simulink model "Single Phase Induction Motor with all methods (final)"  (R2023b)
settings: Solver=ode23s  StartTime=0.0  StopTime=10.0  MaxStep=1e-4  RelTol=1e-3
undefined symbols (not defined in the file): Capacitor, Run, Start
libraries: spsIGBTDiodeLib x12, simulink x9, spsDCVoltageSourceLib x3, spsRMSLib x3, spsSinglePhaseAsynchronousMachineLib x3, spsVoltageMeasurementLib x3, slpidlib x2, spspowerguiLib x2, spsControlledVoltageSourceLib x1, sps_lib x1
settings Model: Creator=Haier  LastModifiedBy=Haier

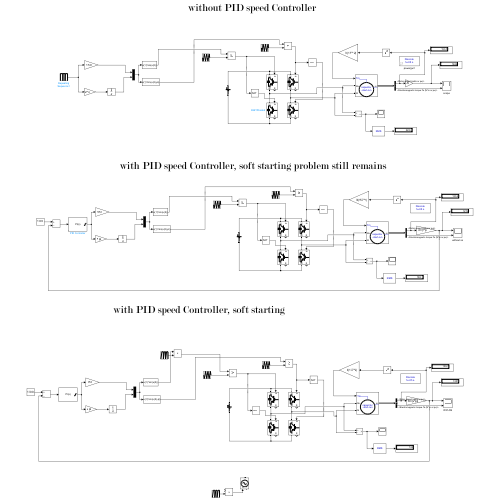
[thumbnail: Simulink's stored preview of the top-level diagram]
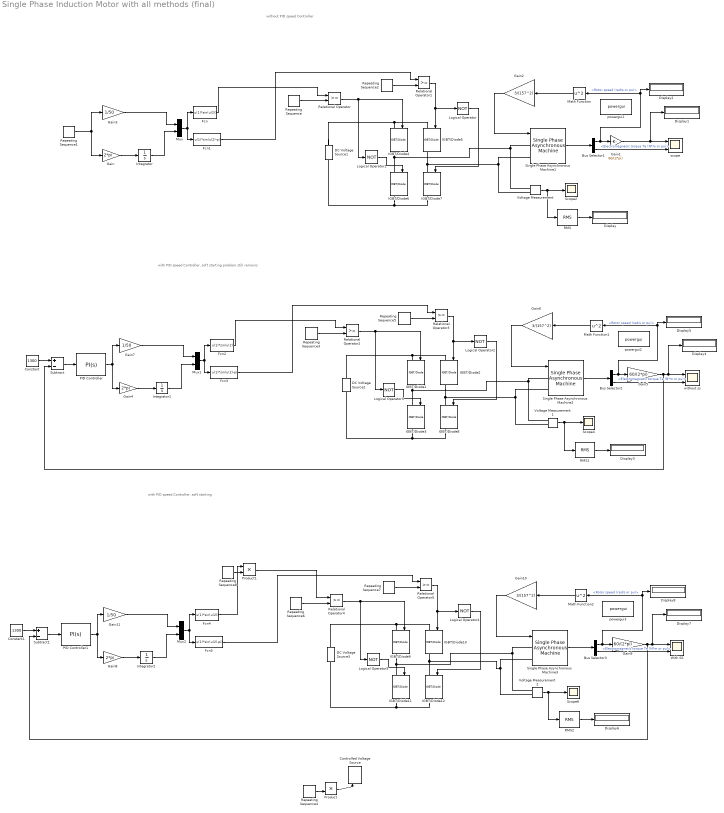
== system Single Phase Induction Motor with all methods (final) ==
  note: without PID speed Controller
  note: with PID speed Controller, soft starting problem still remains
  note: with PID speed Controller, soft starting
  Bus Selector1 : BusSelector  OutputSignals=Mechanical.Rotor speed (rad/s or pu),Mechanical.Electromagnetic torque Te (N*m or pu)
  Bus Selector2 : BusSelector  OutputSignals=Mechanical.Rotor speed (rad/s or pu),Mechanical.Electromagnetic torque Te (N*m or pu)
  Bus Selector3 : BusSelector  OutputSignals=Mechanical.Rotor speed (rad/s or pu),Mechanical.Electromagnetic torque Te (N*m or pu)
  Constant : Constant  Value=1300
  Constant1 : Constant  Value=1300
  Controlled Voltage Source : spsControlledVoltageSourceLib/Controlled Voltage Source  Initialize=on  Source_Type=AC  Amplitude=0  Phase=0  Frequency=0  Measurements=None
  DC Voltage Source1 : spsDCVoltageSourceLib/DC Voltage Source  Amplitude=325  Measurements=None
  DC Voltage Source2 : spsDCVoltageSourceLib/DC Voltage Source  Amplitude=325  Measurements=None
  DC Voltage Source3 : spsDCVoltageSourceLib/DC Voltage Source  Amplitude=325  Measurements=None
  Display{,1..8} (9 alike) : Display
  Fcn : Fcn  Expr=u(1)*sin(u(2))
  Fcn1 : Fcn  Expr=u(1)*sin(u(2)-pi)
  Fcn2 : Fcn  Expr=u(1)*sin(u(2))
  Fcn3 : Fcn  Expr=u(1)*sin(u(2)-pi)
  Fcn4 : Fcn  Expr=u(1)*sin(u(2))
  Fcn5 : Fcn  Expr=u(1)*sin(u(2)-pi)
  Gain : Gain  Gain=2*pi
  Gain1 : Gain  Gain=60/(2*pi)
  Gain10 : Gain  Gain=3/(157^2)
  Gain11 : Gain  Gain=1/50
  Gain2 : Gain  Gain=3/(157^2)
  Gain3 : Gain  Gain=1/50
  Gain4 : Gain  Gain=2*pi
  Gain5 : Gain  Gain=60/(2*pi)
  Gain6 : Gain  Gain=3/(157^2)
  Gain7 : Gain  Gain=1/50
  Gain8 : Gain  Gain=2*pi
  Gain9 : Gain  Gain=60/(2*pi)
  IGBT/Diode{1..12} (12 alike) : spsIGBTDiodeLib/IGBT//Diode  Ron=1e-3  Rs=1e5  Cs=inf  Measurements=on
  Integrator : Integrator
  Integrator1 : Integrator
  Integrator2 : Integrator
  Logical Operator{,1..5} (6 alike) : Logic  Operator=NOT  AllPortsSameDT=off  OutDataTypeStr=boolean
  Math Function : Math  Operator=square
  Math Function1 : Math  Operator=square
  Math Function2 : Math  Operator=square
  Mux : Mux  Inputs=2
  Mux1 : Mux  Inputs=2
  Mux2 : Mux  Inputs=2
  PID Controller : slpidlib/PID Controller  Controller=PI  Form=Parallel  TimeDomain=Continuous-time  UseExternalTs=off  SampleTime=-1  IntegratorMethod=Forward Euler  FilterMethod=Forward Euler  ControllerParametersSource=internal  P=0.00001  I=0.09  UseKiTs=off  D=0  N=100  UseFilter=on  TunerSelectOption=Transfer Function Based (PID Tuner App)  InitialConditionSource=internal  InitialConditionForIntegrator=0  InitialConditionForFilter=0  DifferentiatorICPrevScaledInput=0  ExternalReset=none  TrackingMode=off  Kt=1  LimitOutput=on  SatLimitsSource=internal  UpperSaturationLimit=50  LowerSaturationLimit=-50  LinearizeAsGain=on  AntiWindupMode=clamping  Kb=1  LimitIntegrator=off  UpperIntegratorSaturationLimit=inf  LowerIntegratorSaturationLimit=-inf  POutMin=[]  POutMax=[]  IOutMin=[]  IOutMax=[]  DOutMin=[]  DOutMax=[]  NOutMin=[]  NOutMax=[]  SumOutMin=[]  SumOutMax=[]  SaturationOutMin=[]  SaturationOutMax=[]  PParamMin=[]  PParamMax=[]  IParamMin=[]  IParamMax=[]  DParamMin=[]  DParamMax=[]  NParamMin=[]  NParamMax=[]  KbParamMin=[]  KbParamMax=[]  KtParamMin=[]  KtParamMax=[]  KbOutMin=[]  KbOutMax=[]  KtOutMin=[]  KtOutMax=[]  IntegratorOutMin=[]  IntegratorOutMax=[]  FilterOutMin=[]  FilterOutMax=[]  SumI1OutMin=[]  SumI1OutMax=[]  SumI2OutMin=[]  SumI2OutMax=[]  SumI3OutMin=[]  SumI3OutMax=[]  SumI4OutMin=[]  SumI4OutMax=[]  SumDOutMin=[]  SumDOutMax=[]  DifferentiatorOutMin=[]  DifferentiatorOutMax=[]  FilterDiffOutCoefMin=[]  FilterDiffOutCoefMax=[]  ReciprocalOutMin=[]  ReciprocalOutMax=[]  SumDenOutMin=[]  SumDenOutMax=[]  SumNumOutMin=[]  SumNumOutMax=[]  DivideOutMin=[]  DivideOutMax=[]  UdiffTsProdOutMin=[]  UdiffTsProdOutMax=[]  NTsProdOutMin=[]  NTsProdOutMax=[]  UintegralTsProdOutMin=[]  UintegralTsProdOutMax=[]  UngainTsProdOutMin=[]  UngainTsProdOutMax=[]  ClampingZeroOutDataTypeStr=Inherit: Inherit via back propagation  ClampingZeroOutMin=[]  ClampingZeroOutMax=[]  FilterDenConstantOutDataTypeStr=Inherit: Inherit via back propagation  FilterDenConstantOutMin=[]  FilterDenConstantOutMax=[]  PCopyOutDataTypeStr=Inherit: Inherit via back propagation  PCopyOutMin=[]  PCopyOutMax=[]  NCopyOutDataTypeStr=Inherit: Inherit via back propagation  NCopyOutMin=[]  NCopyOutMax=[]  IntegratorContinuousStateAttributes=''  IntegratorStateMustResolveToSignalObject=off  IntegratorRTWStateStorageClass=Auto  FilterContinuousStateAttributes=''  FilterStateMustResolveToSignalObject=off  FilterRTWStateStorageClass=Auto  ParallelPVariant=InternalParameters  IdealPVariant=Disabled  IVariant=InternalParameters  DVariant=Disabled  IntegratorVariant=Continuous  SatVariant=Enabled  AWVariant=ContClampingParallel  PCopyVariant=Disabled  TRVariant=Disabled  FdbkBlocksVariant=Forward  IdealPFdbkVariant=Disabled  SatFdbkVariant=Disabled  DerivativeFilterVariant=Disabled  NVariant=Disabled  NCopyVariant=Disabled_SignalSpec  FilterICVariant=Disabled  IntegratorICVariant=InternalICs  ExternalResetVariant=Disabled  TRSumVariant=Passthrough  SumFdbkVariant=Disabled  SumVariant=Sum_PI  TsampFilterVariant=InternalTs  TsampNgainVariant=Passthrough  TsampIntegralVariant=Disabled_SignalSpec  ExternalSaturationOutDataTypeStr=Inherit: Same as second input
  PID Controller1 : slpidlib/PID Controller  Controller=PI  Form=Parallel  TimeDomain=Continuous-time  UseExternalTs=off  SampleTime=-1  IntegratorMethod=Forward Euler  FilterMethod=Forward Euler  ControllerParametersSource=internal  P=0.00001  I=0.09  UseKiTs=off  D=0  N=100  UseFilter=on  TunerSelectOption=Transfer Function Based (PID Tuner App)  InitialConditionSource=internal  InitialConditionForIntegrator=0  InitialConditionForFilter=0  DifferentiatorICPrevScaledInput=0  ExternalReset=none  TrackingMode=off  Kt=1  LimitOutput=on  SatLimitsSource=internal  UpperSaturationLimit=50  LowerSaturationLimit=-50  LinearizeAsGain=on  AntiWindupMode=clamping  Kb=1  LimitIntegrator=off  UpperIntegratorSaturationLimit=inf  LowerIntegratorSaturationLimit=-inf  POutMin=[]  POutMax=[]  IOutMin=[]  IOutMax=[]  DOutMin=[]  DOutMax=[]  NOutMin=[]  NOutMax=[]  SumOutMin=[]  SumOutMax=[]  SaturationOutMin=[]  SaturationOutMax=[]  PParamMin=[]  PParamMax=[]  IParamMin=[]  IParamMax=[]  DParamMin=[]  DParamMax=[]  NParamMin=[]  NParamMax=[]  KbParamMin=[]  KbParamMax=[]  KtParamMin=[]  KtParamMax=[]  KbOutMin=[]  KbOutMax=[]  KtOutMin=[]  KtOutMax=[]  IntegratorOutMin=[]  IntegratorOutMax=[]  FilterOutMin=[]  FilterOutMax=[]  SumI1OutMin=[]  SumI1OutMax=[]  SumI2OutMin=[]  SumI2OutMax=[]  SumI3OutMin=[]  SumI3OutMax=[]  SumI4OutMin=[]  SumI4OutMax=[]  SumDOutMin=[]  SumDOutMax=[]  DifferentiatorOutMin=[]  DifferentiatorOutMax=[]  FilterDiffOutCoefMin=[]  FilterDiffOutCoefMax=[]  ReciprocalOutMin=[]  ReciprocalOutMax=[]  SumDenOutMin=[]  SumDenOutMax=[]  SumNumOutMin=[]  SumNumOutMax=[]  DivideOutMin=[]  DivideOutMax=[]  UdiffTsProdOutMin=[]  UdiffTsProdOutMax=[]  NTsProdOutMin=[]  NTsProdOutMax=[]  UintegralTsProdOutMin=[]  UintegralTsProdOutMax=[]  UngainTsProdOutMin=[]  UngainTsProdOutMax=[]  ClampingZeroOutDataTypeStr=Inherit: Inherit via back propagation  ClampingZeroOutMin=[]  ClampingZeroOutMax=[]  FilterDenConstantOutDataTypeStr=Inherit: Inherit via back propagation  FilterDenConstantOutMin=[]  FilterDenConstantOutMax=[]  PCopyOutDataTypeStr=Inherit: Inherit via back propagation  PCopyOutMin=[]  PCopyOutMax=[]  NCopyOutDataTypeStr=Inherit: Inherit via back propagation  NCopyOutMin=[]  NCopyOutMax=[]  IntegratorContinuousStateAttributes=''  IntegratorStateMustResolveToSignalObject=off  IntegratorRTWStateStorageClass=Auto  FilterContinuousStateAttributes=''  FilterStateMustResolveToSignalObject=off  FilterRTWStateStorageClass=Auto  ParallelPVariant=InternalParameters  IdealPVariant=Disabled  IVariant=InternalParameters  DVariant=Disabled  IntegratorVariant=Continuous  SatVariant=Enabled  AWVariant=ContClampingParallel  PCopyVariant=Disabled  TRVariant=Disabled  FdbkBlocksVariant=Forward  IdealPFdbkVariant=Disabled  SatFdbkVariant=Disabled  DerivativeFilterVariant=Disabled  NVariant=Disabled  NCopyVariant=Disabled_SignalSpec  FilterICVariant=Disabled  IntegratorICVariant=InternalICs  ExternalResetVariant=Disabled  TRSumVariant=Passthrough  SumFdbkVariant=Disabled  SumVariant=Sum_PI  TsampFilterVariant=InternalTs  TsampNgainVariant=Passthrough  TsampIntegralVariant=Disabled_SignalSpec  ExternalSaturationOutDataTypeStr=Inherit: Same as second input
  Product : Product
  Product1 : Product
  RMS : spsRMSLib/RMS  TrueRMS=off  Freq=50  RMSInit=0  Ts=0
  RMS1 : spsRMSLib/RMS  TrueRMS=off  Freq=50  RMSInit=0  Ts=0
  RMS2 : spsRMSLib/RMS  TrueRMS=off  Freq=50  RMSInit=0  Ts=0
  Relational Operator{,1..5} (6 alike) : RelationalOperator  OutDataTypeStr=boolean  RndMeth=Simplest  InputSameDT=off
  Repeating Sequence{,2..3,5..7} (6 alike) : simulink/Sources/Repeating Sequence  rep_seq_t=[0 0.25/5000 0.5/5000 0.75/5000 1/5000]  rep_seq_y=[0 -1 0 1 0]
  Repeating Sequence1 : simulink/Sources/Repeating Sequence  rep_seq_t=[0 0.2 10]  rep_seq_y=[0 50 50]
  Repeating Sequence4 : simulink/Sources/Repeating Sequence  rep_seq_t=[0 4 10]  rep_seq_y=[0 1 1]
  Repeating Sequence8 : simulink/Sources/Repeating Sequence  rep_seq_t=[0 4 10]  rep_seq_y=[0 1 1]
  Scope2 : Scope
  Scope4 : Scope
  Scope6 : Scope
  Single Phase Asynchronous Machine1 : spsSinglePhaseAsynchronousMachineLib/Single Phase Asynchronous Machine  MechanicalLoad=Torque Tm  UNITS=SI  MachineType=Capacitor-Start-Run  MeasurementBus=off  NominalParameters="[ .25*746  220  50]"  MainWindingStator="[2.02  7.4e-3]"  MainWindingRotor="[4.12  5.6e-3]"  MutualInductance=0.1772  AuxiliaryWinding="[7.14  8.5e-3]"  Mechanical="[0.0146  0  2 1.18]"  CapacitorStart="[2  254.7e-6]"  CapacitorRun="[18  21.1e-6]"  DisconnectionSpeed=75  InitialSpeed=0  DataType=SI  TsPowergui=0  TsBlock=-1
      settings: LibrarySourceBlock=|
      | sps_lib/Electrical Machines/Single Phase
      | Asynchronous Machine
  Single Phase Asynchronous Machine2 : spsSinglePhaseAsynchronousMachineLib/Single Phase Asynchronous Machine  MechanicalLoad=Torque Tm  UNITS=SI  MachineType=Capacitor-Start-Run  MeasurementBus=off  NominalParameters="[ .25*746  220  50]"  MainWindingStator="[2.02  7.4e-3]"  MainWindingRotor="[4.12  5.6e-3]"  MutualInductance=0.1772  AuxiliaryWinding="[7.14  8.5e-3]"  Mechanical="[0.0146  0  2 1.18]"  CapacitorStart="[2  254.7e-6]"  CapacitorRun="[18  21.1e-6]"  DisconnectionSpeed=75  InitialSpeed=0  DataType=SI  TsPowergui=0  TsBlock=-1
      settings: LibrarySourceBlock=|
      | sps_lib/Electrical Machines/Single Phase
      | Asynchronous Machine
  Single Phase Asynchronous Machine3 : spsSinglePhaseAsynchronousMachineLib/Single Phase Asynchronous Machine  MechanicalLoad=Torque Tm  UNITS=SI  MachineType=Capacitor-Start-Run  MeasurementBus=off  NominalParameters="[ .25*746  220  50]"  MainWindingStator="[2.02  7.4e-3]"  MainWindingRotor="[4.12  5.6e-3]"  MutualInductance=0.1772  AuxiliaryWinding="[7.14  8.5e-3]"  Mechanical="[0.0146  0  2 1.18]"  CapacitorStart="[2  254.7e-6]"  CapacitorRun="[18  21.1e-6]"  DisconnectionSpeed=75  InitialSpeed=0  DataType=SI  TsPowergui=0  TsBlock=-1
      settings: LibrarySourceBlock=|
      | sps_lib/Electrical Machines/Single Phase
      | Asynchronous Machine
  Subtract : Sum  Inputs=+-
  Subtract1 : Sum  Inputs=+-
  Voltage Measurement : spsVoltageMeasurementLib/Voltage Measurement  PhasorSimulation=off  OutputType=Complex  PSBequivalent=0
  Voltage Measurement1 : spsVoltageMeasurementLib/Voltage Measurement  PhasorSimulation=off  OutputType=Complex  PSBequivalent=0
  Voltage Measurement2 : spsVoltageMeasurementLib/Voltage Measurement  PhasorSimulation=off  OutputType=Complex  PSBequivalent=0
  With SS : Scope  NumInputPorts=2
  powergui1 : sps_lib/powergui  Priority=1  SimulationMode=Discrete  SampleTime=1e-5  frequency=60  Iterations=50  frequencyindice=0  Pbase=100e6  ErrMax=1e-4  UnitsV=kV  UnitsW=MW  buscounter=0  FunctionMessages=off  echomessages=off  EnableUseOfTLC=off  CurrentSourceSwitches=off  DisableSnubberDevices=off  DisableRonSwitches=off  DisableVfSwitches=off  DisplayEquations=off  AutomaticDiscreteSolvers=off  SolverType=Tustin/Backward Euler (TBE)  Interpol=off  ExternalGateDelay=off  methode=off  Ts=100  x0status=blocks  SPID=on  SwTol=0  HookPort=off  NonlinearTolerance=1e-4  nMaxIteration=100  ContinueOnMaxIteration=off  RestoreLinks=warning  ResistiveCurrentMeasurement=off  Frange=[0:2:500]  Ylog=off  Xlog=on  ShowGrid=off  save=off  variable=ZData  structure=0  ZoomFFT=off  StartTime=0.0  cycles=1  DisplayStyle=1  fundamental=60  FreqAxis=off  MaxFrequency=1000  frequencyindicesteady=1  RmsSteady=1  display=off
  powergui2 : spspowerguiLib/powergui  Priority=1  SimulationMode=Discrete  SampleTime=1e-5  frequency=60  Iterations=50  frequencyindice=0  Pbase=100e6  ErrMax=1e-4  UnitsV=kV  UnitsW=MW  buscounter=0  FunctionMessages=off  echomessages=off  EnableUseOfTLC=off  CurrentSourceSwitches=off  DisableSnubberDevices=off  DisableRonSwitches=off  DisableVfSwitches=off  DisplayEquations=off  AutomaticDiscreteSolvers=off  SolverType=Tustin/Backward Euler (TBE)  Interpol=off  ExternalGateDelay=off  methode=off  Ts=100  x0status=blocks  SPID=on  SwTol=0  HookPort=off  NonlinearTolerance=1e-4  nMaxIteration=100  ContinueOnMaxIteration=off  RestoreLinks=warning  ResistiveCurrentMeasurement=off  Frange=[0:2:500]  Ylog=off  Xlog=on  ShowGrid=off  save=off  variable=ZData  structure=0  ZoomFFT=off  StartTime=0.0  cycles=1  DisplayStyle=1  fundamental=60  FreqAxis=off  MaxFrequency=1000  frequencyindicesteady=1  RmsSteady=1  display=off
  powergui3 : spspowerguiLib/powergui  Priority=1  SimulationMode=Discrete  SampleTime=1e-5  frequency=60  Iterations=50  frequencyindice=0  Pbase=100e6  ErrMax=1e-4  UnitsV=kV  UnitsW=MW  buscounter=0  FunctionMessages=off  echomessages=off  EnableUseOfTLC=off  CurrentSourceSwitches=off  DisableSnubberDevices=off  DisableRonSwitches=off  DisableVfSwitches=off  DisplayEquations=off  AutomaticDiscreteSolvers=off  SolverType=Tustin/Backward Euler (TBE)  Interpol=off  ExternalGateDelay=off  methode=off  Ts=100  x0status=blocks  SPID=on  SwTol=0  HookPort=off  NonlinearTolerance=1e-4  nMaxIteration=100  ContinueOnMaxIteration=off  RestoreLinks=warning  ResistiveCurrentMeasurement=off  Frange=[0:2:500]  Ylog=off  Xlog=on  ShowGrid=off  save=off  variable=ZData  structure=0  ZoomFFT=off  StartTime=0.0  cycles=1  DisplayStyle=1  fundamental=60  FreqAxis=off  MaxFrequency=1000  frequencyindicesteady=1  RmsSteady=1  display=off
  scope : Scope  NumInputPorts=2
  without ss : Scope  NumInputPorts=2
  wires:
  Bus Selector1/1 -> Math Function/1, Display2/1, Gain1/1  "<Rotor speed (rad/s or pu)>"
  Voltage Measurement/1 -> RMS/1, Scope2/1
  Gain1/1 -> Display1/1, scope/1
  Math Function/1 -> Gain2/1
  Gain2/1 -> Single Phase Asynchronous Machine1/1
  Single Phase Asynchronous Machine1/1 -> Bus Selector1/1
  Bus Selector1/2 -> scope/2  "<Electromagnetic torque Te (N*m or pu)>"
  Integrator/1 -> Mux/2
  Gain3/1 -> Mux/1
  Mux/1 -> Fcn1/1, Fcn/1
  Gain/1 -> Integrator/1
  Repeating Sequence1/1 -> Gain/1, Gain3/1
  RMS/1 -> Display/1
  Relational Operator1/1 -> IGBT/Diode5/1, Logical Operator/1
  Relational Operator/1 -> Logical Operator1/1, IGBT/Diode4/1
  Logical Operator1/1 -> IGBT/Diode6/1
  Logical Operator/1 -> IGBT/Diode7/1
  Repeating Sequence/1 -> Relational Operator/2
  Repeating Sequence2/1 -> Relational Operator1/2
  Fcn/1 -> Relational Operator/1
  Fcn1/1 -> Relational Operator1/1
  Gain4/1 -> Integrator1/1
  Integrator1/1 -> Mux1/2
  Repeating Sequence5/1 -> Relational Operator3/2
  Relational Operator3/1 -> IGBT/Diode2/1, Logical Operator2/1
  Fcn2/1 -> Relational Operator2/1
  Fcn3/1 -> Relational Operator3/1
  Logical Operator3/1 -> IGBT/Diode3/1
  Gain7/1 -> Mux1/1
  Relational Operator2/1 -> Logical Operator3/1, IGBT/Diode1/1
  Repeating Sequence3/1 -> Relational Operator2/2
  Mux1/1 -> Fcn3/1, Fcn2/1
  Gain6/1 -> Single Phase Asynchronous Machine2/1
  Single Phase Asynchronous Machine2/1 -> Bus Selector2/1
  Math Function1/1 -> Gain6/1
  Voltage Measurement1/1 -> RMS1/1, Scope4/1
  Bus Selector2/1 -> Math Function1/1, Display5/1, Gain5/1  "<Rotor speed (rad/s or pu)>"
  Bus Selector2/2 -> without ss/2  "<Electromagnetic torque Te (N*m or pu)>"
  RMS1/1 -> Display3/1
  Logical Operator2/1 -> IGBT/Diode8/1
  Constant/1 -> Subtract/1
  Gain5/1 -> Subtract/2, Display4/1, without ss/1
  PID Controller/1 -> Gain4/1, Gain7/1
  Subtract/1 -> PID Controller/1
  Subtract1/1 -> PID Controller1/1
  Bus Selector3/1 -> Math Function2/1, Display8/1, Gain9/1  "<Rotor speed (rad/s or pu)>"
  Math Function2/1 -> Gain10/1
  Single Phase Asynchronous Machine3/1 -> Bus Selector3/1
  Bus Selector3/2 -> With SS/2  "<Electromagnetic torque Te (N*m or pu)>"
  Mux2/1 -> Fcn5/1, Fcn4/1
  Relational Operator4/1 -> Logical Operator5/1, IGBT/Diode9/1
  Logical Operator5/1 -> IGBT/Diode11/1
  Fcn5/1 -> Relational Operator5/1
  Gain11/1 -> Mux2/1
  Relational Operator5/1 -> IGBT/Diode10/1, Logical Operator4/1
  Repeating Sequence6/1 -> Relational Operator4/2
  Repeating Sequence7/1 -> Relational Operator5/2
  Integrator2/1 -> Mux2/2
  Gain8/1 -> Integrator2/1
  Gain9/1 -> Subtract1/2, Display7/1, With SS/1
  Gain10/1 -> Single Phase Asynchronous Machine3/1
  Voltage Measurement2/1 -> RMS2/1, Scope6/1
  PID Controller1/1 -> Gain8/1, Gain11/1
  Constant1/1 -> Subtract1/1
  RMS2/1 -> Display6/1
  Logical Operator4/1 -> IGBT/Diode12/1
  Product/1 -> Controlled Voltage Source/1
  Repeating Sequence4/1 -> Product/2
  Repeating Sequence8/1 -> Product1/2
  Fcn4/1 -> Product1/1
  Product1/1 -> Relational Operator4/1
  connections:
  DC Voltage Source1/RConn1 -- IGBT/Diode4/LConn1 -- IGBT/Diode5/LConn1
  IGBT/Diode6/RConn1 -- IGBT/Diode7/RConn1 -- DC Voltage Source1/LConn1
  Voltage Measurement/LConn1 -- IGBT/Diode6/LConn1 -- IGBT/Diode4/RConn1 -- Single Phase Asynchronous Machine1/LConn1
  IGBT/Diode5/RConn1 -- Voltage Measurement/LConn2 -- Single Phase Asynchronous Machine1/LConn2 -- IGBT/Diode7/LConn1
  IGBT/Diode1/RConn1 -- Single Phase Asynchronous Machine2/LConn1 -- Voltage Measurement1/LConn1 -- IGBT/Diode3/LConn1
  IGBT/Diode2/LConn1 -- IGBT/Diode1/LConn1 -- DC Voltage Source2/RConn1
  IGBT/Diode2/RConn1 -- Voltage Measurement1/LConn2 -- Single Phase Asynchronous Machine2/LConn2 -- IGBT/Diode8/LConn1
  IGBT/Diode3/RConn1 -- IGBT/Diode8/RConn1 -- DC Voltage Source2/LConn1
  Single Phase Asynchronous Machine3/LConn2 -- IGBT/Diode12/LConn1 -- IGBT/Diode10/RConn1 -- Voltage Measurement2/LConn2
  IGBT/Diode11/RConn1 -- IGBT/Diode12/RConn1 -- DC Voltage Source3/LConn1
  Voltage Measurement2/LConn1 -- IGBT/Diode9/RConn1 -- IGBT/Diode11/LConn1 -- Single Phase Asynchronous Machine3/LConn1
  IGBT/Diode9/LConn1 -- IGBT/Diode10/LConn1 -- DC Voltage Source3/RConn1
